simulink model "system"  (R2020b)
settings: Solver=VariableStepAuto  StartTime=0.0  StopTime=10.0  RelTol=1e-3
values from neighbouring files (symbols this model uses):
  E0 = 0.145    [simulation.m]
  I0 = 0.05    [simulation.m]
  J0 = 0.005    [simulation.m]
  S0 = 0.8    [simulation.m]
settings Model: Creator=leumas  LastModifiedBy=leumas

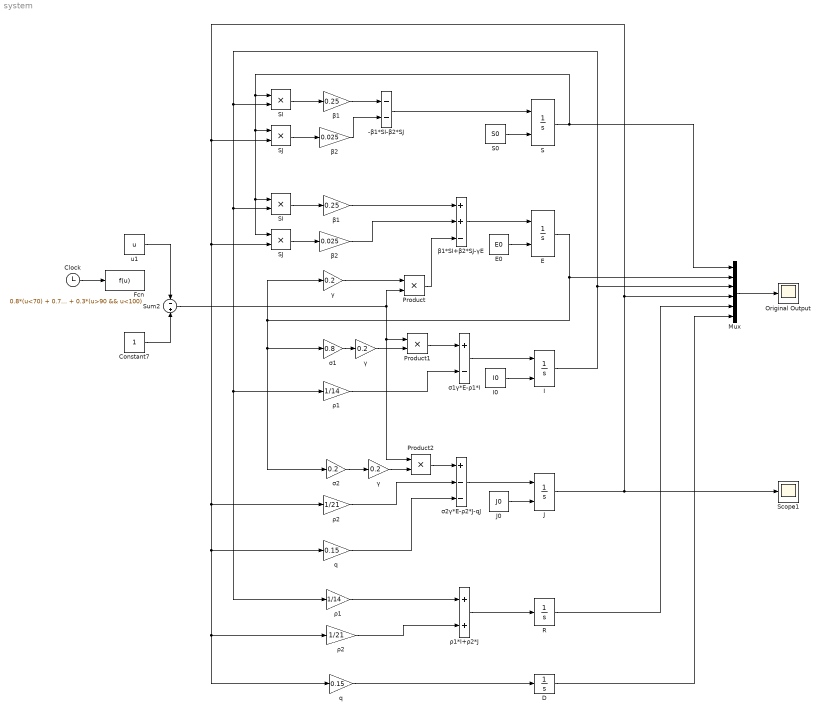
== system system ==
  -β1*SI-β2*SJ : Sum  Inputs=--
  Clock : Clock
  Constant7 : Constant
  D : Integrator
  E : Integrator  InitialConditionSource=external
  E0 : Constant  Value=E0
  Fcn : Fcn  Expr=0.8*(u<70) + 0.7*(u>70 && u<90) + 0.3*(u>90 && u<100)
  I : Integrator  InitialConditionSource=external
  I0 : Constant  Value=I0
  J : Integrator  InitialConditionSource=external
  J0 : Constant  Value=J0
  Mux : Mux  Inputs=6
  Original Output : Scope
  Product : Product
  Product1 : Product
  Product2 : Product
  R : Integrator
  S : Integrator  InitialConditionSource=external
  S0 : Constant  Value=S0
  SI : Product
  "SI " : Product
  SJ : Product
  "SJ " : Product
  Scope1 : Scope
  Sum2 : Sum  Inputs=-+
  q : Gain  Gain=0.15
  "q " : Gain  Gain=0.15
  u1 : Constant  Value=u
  β1 : Gain  Gain=0.25
  "β1   " : Gain  Gain=0.25
  β1*SI+β2*SJ-γE : Sum  Inputs=++-
  β2 : Gain  Gain=0.025
  "β2 " : Gain  Gain=0.025
  γ : Gain  Gain=0.2
  "γ " : Gain  Gain=0.2
  "γ  " : Gain  Gain=0.2
  ρ1 : Gain  Gain=1/14
  "ρ1 " : Gain  Gain=1/14
  ρ1*I+ρ2*J : Sum
  ρ2 : Gain  Gain=1/21
  "ρ2 " : Gain  Gain=1/21
  σ1 : Gain  Gain=0.8
  σ1γ*E-ρ1*I : Sum  Inputs=+-
  σ2 : Gain  Gain=0.2
  σ2γ*E-ρ2*J-qJ : Sum  Inputs=+--
  wires:
  u1/1 -> Sum2/1
  J/1 -> Scope1/1, q/1, "q "/1, "ρ2 "/1, ρ2/1, "SJ "/2, SJ/2, Mux/4
  "γ "/1 -> Product2/2
  Constant7/1 -> Sum2/2
  Clock/1 -> Fcn/1
  I/1 -> ρ1/1, "ρ1 "/1, "SI "/2, SI/2, Mux/3
  -β1*SI-β2*SJ/1 -> S/1
  E0/1 -> E/2
  β2/1 -> -β1*SI-β2*SJ/2
  SJ/1 -> β2/1
  β1/1 -> -β1*SI-β2*SJ/1
  Product2/1 -> σ2γ*E-ρ2*J-qJ/1
  "β2 "/1 -> β1*SI+β2*SJ-γE/2
  "γ  "/1 -> Product1/2
  S/1 -> "SJ "/1, "SI "/1, SJ/1, SI/1, Mux/1
  J0/1 -> J/2
  SI/1 -> β1/1
  σ1γ*E-ρ1*I/1 -> I/1
  σ1/1 -> "γ  "/1
  σ2/1 -> "γ "/1
  "SI "/1 -> "β1   "/1
  ρ2/1 -> σ2γ*E-ρ2*J-qJ/2
  Sum2/1 -> Product1/1, Product2/1, Product/2
  ρ1/1 -> σ1γ*E-ρ1*I/2
  "q "/1 -> D/1
  "ρ1 "/1 -> ρ1*I+ρ2*J/1
  "ρ2 "/1 -> ρ1*I+ρ2*J/2
  ρ1*I+ρ2*J/1 -> R/1
  "SJ "/1 -> "β2 "/1
  σ2γ*E-ρ2*J-qJ/1 -> J/1
  R/1 -> Mux/5
  Mux/1 -> Original Output/1
  D/1 -> Mux/6
  γ/1 -> Product/1
  Product1/1 -> σ1γ*E-ρ1*I/1
  q/1 -> σ2γ*E-ρ2*J-qJ/3
  S0/1 -> S/2
  β1*SI+β2*SJ-γE/1 -> E/1
  I0/1 -> I/2
  "β1   "/1 -> β1*SI+β2*SJ-γE/1
  E/1 -> γ/1, σ2/1, σ1/1, Mux/2
  Product/1 -> β1*SI+β2*SJ-γE/3
